simulink model "analise_de_resposta_transitoria"  (R2023a)
settings: Solver=VariableStepAuto  StartTime=0.0  StopTime=5  RelTol=1e-3
settings Model: Creator=stem  LastModifiedBy=stem

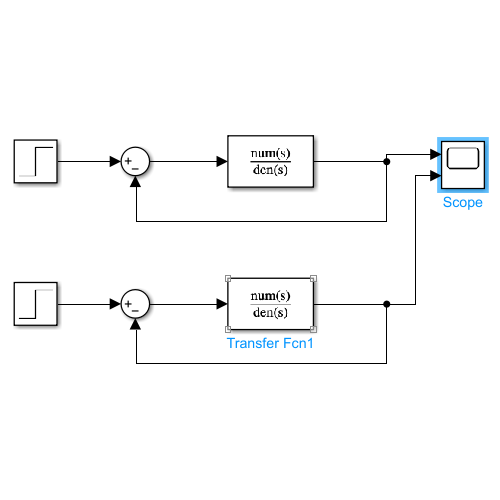
[thumbnail: Simulink's stored preview of the top-level diagram]
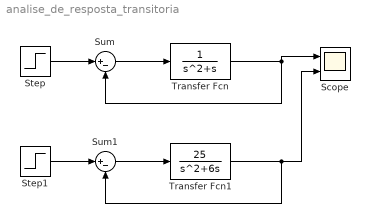
== system analise_de_resposta_transitoria ==
  Scope : Scope  NumInputPorts=2
  Step : Step  Before=1  SampleTime=0
  Step1 : Step  Before=1  SampleTime=0
  Sum : Sum  Inputs=|+-
  Sum1 : Sum  Inputs=|+-
  Transfer Fcn : TransferFcn  Denominator=[1 1 0]
  Transfer Fcn1 : TransferFcn  Numerator=[25]  Denominator=[1 6 0]
  wires:
  Transfer Fcn/1 -> Scope/1, Sum/2
  Step/1 -> Sum/1
  Sum/1 -> Transfer Fcn/1
  Transfer Fcn1/1 -> Scope/2, Sum1/2
  Sum1/1 -> Transfer Fcn1/1
  Step1/1 -> Sum1/1
